simulink model "tqdtqr_rebuild_V3"  (R2021b)
settings: Solver=VariableStepAuto  StartTime=0.0  StopTime=10.0  RelTol=1e-3
undefined symbols (not defined in the file): ATQD_AfterTqMinGain_X_Deg, ATQD_APSCreepBaseTqD_X_kph, ATQD_APSCreepBaseTqD_Y_Deg, ATQD_APSCreepBaseTqR_X_kph, ATQD_APSCreepBaseTqR_Y_Deg, ATQD_APSCreepIterm_X_kph, ATQD_APSCreepIterm_Y_kph, ATQD_APSCreepPterm_X_kph, ATQD_APSCreepPterm_Y_kph, ATQD_APSDecReq_X_kph, ATQD_APSDecReq_Y_mps2, ATQD_APSDecReqCMD_X_kph, ATQD_APSDecReqTs_X_pct, ATQD_APSDecTimeGain_X_Deg, ATQD_APSDecTimeGain_Y_s, ATQD_APSReqLowSpd_X_Deg, ATQD_AutoHoldReleaseBPS_X_Deg, ATQD_AWDLoadTrqnsGain_X_kg, ATQD_AWDLoadTrqnsGain_Y_pct, ATQD_BOSEnBPSPosn_X_kph, ATQD_BOSMap_X_rpm, ATQD_BOSMap_Y_pct, ATQD_CreepBaseTqD_X_kph, ATQD_CreepBaseTqD_Y_Deg, ATQD_CreepBaseTqR_X_kph, ATQD_CreepBaseTqR_Y_Deg, ATQD_CreepBPSDisPosn_X_Deg, ATQD_CreepBPSDisPosnR_X_Deg, ATQD_CreepBPSEnPosn_X_Deg, ATQD_CreepBPSEnPosnR_X_Deg, ATQD_CreepDeltaTq_X_kph, ATQD_CreepIterm_X_kph, ATQD_CreepIterm_Y_kph, ATQD_CreepItermMaxLimit_X_pct, ATQD_CreepPreloadTime_X_kph, ATQD_CreepPreloadTq_X_kph, ATQD_CreepPreloadTq_Y_s, ATQD_CreepProtTq_X_Deg, ATQD_CreepPterm_X_kph, ATQD_CreepPterm_Y_kph, ATQD_CreepRrTqSpRat_X_rpm, ATQD_CreepRrTqSpRat_Y_Nm, ATQD_CreepTargetSpdD_X_pct, ATQD_CreepTargetSpdR_X_pct, ATQD_CreepUpLimitTq_X_rpm, ATQD_DecIneOPDHoldEnDelay_X_Deg, ATQD_DecIneOPDHoldEnDelay_Y_bar, ATQD_ECOTqMapD_X_rpm, ATQD_ECOTqMapD_Y_pct, ATQD_EMTqMapD_X_rpm, ATQD_EMTqMapD_Y_pct, ATQD_EOPDTqMapDCon_X_rpm, ATQD_EOPDTqMapDCon_Y_Deg, ATQD_EstInitVehWeight_X_c, ATQD_FAfterTqCMDGain_X_rpm, ATQD_FAfterTqCMDGain_Y_pct, ATQD_ForceLowSpd_X_Deg, ATQD_ForcePLimitSpd_X_Deg, ATQD_FrLossMAPLowV_X_rpm, ATQD_FrLossMAPLowV_Y_Nm ... (+949)
libraries: simulink x235, hcu_lib x208, tqr x63, tqd x6
(part 34 of 37)

== system tqdtqr_rebuild_V3/Input_Convert/Signal function/combo key/Combo Key Detection/Engineering Mode/Key3/Reset ==
  Action Port : ActionPort  ActionPortLabel=if(u1 ~=0)
  Constant : Constant  Value=ENUM_COMBOKEY_NONE
  ResetToZero : Outport
  wires:
  Constant/1 -> ResetToZero/1

== system tqdtqr_rebuild_V3/Input_Convert/Signal function/combo key/Combo Key Detection/Engineering Mode/Key3/Write ==
  Input : Inport
  Action Port : ActionPort  ActionPortLabel=elseif(u2 ~= 0)
  WriteCMD : Outport
  wires:
  Input/1 -> WriteCMD/1

== system tqdtqr_rebuild_V3/Input_Convert/Signal function/combo key/Combo Key Detection/Engineering Mode/Key4/Maintain ==
  Input : Inport
  Action Port : ActionPort  ActionPortLabel=else
  KeepKey4 : Outport
  wires:
  Input/1 -> KeepKey4/1

== system tqdtqr_rebuild_V3/Input_Convert/Signal function/combo key/Combo Key Detection/Engineering Mode/Key4/Reset ==
  Action Port : ActionPort  ActionPortLabel=if(u1 ~=0)
  Constant : Constant  Value=ENUM_COMBOKEY_NONE
  ResetToZero : Outport
  wires:
  Constant/1 -> ResetToZero/1

== system tqdtqr_rebuild_V3/Input_Convert/Signal function/combo key/Combo Key Detection/Engineering Mode/Key4/Write ==
  Input : Inport
  Action Port : ActionPort  ActionPortLabel=elseif(u2 ~= 0)
  WriteCMD : Outport
  wires:
  Input/1 -> WriteCMD/1

== system tqdtqr_rebuild_V3/Input_Convert/Signal function/combo key/Combo Key Detection/Engineering Mode/Key5/Maintain ==
  Input : Inport
  Action Port : ActionPort  ActionPortLabel=else
  KeepKey5 : Outport
  wires:
  Input/1 -> KeepKey5/1

== system tqdtqr_rebuild_V3/Input_Convert/Signal function/combo key/Combo Key Detection/Engineering Mode/Key5/Reset ==
  Action Port : ActionPort  ActionPortLabel=if(u1 ~=0)
  Constant : Constant  Value=ENUM_COMBOKEY_NONE
  ResetToZero : Outport
  wires:
  Constant/1 -> ResetToZero/1

== system tqdtqr_rebuild_V3/Input_Convert/Signal function/combo key/Combo Key Detection/Engineering Mode/Key5/Write ==
  Input : Inport
  Action Port : ActionPort  ActionPortLabel=elseif(u2 ~= 0)
  WriteCMD : Outport
  wires:
  Input/1 -> WriteCMD/1

== system tqdtqr_rebuild_V3/Input_Convert/Signal function/combo key/Combo Key Detection/Engineering Mode/Key6/Maintain ==
  Input : Inport
  Action Port : ActionPort  ActionPortLabel=else
  KeepKey6 : Outport
  wires:
  Input/1 -> KeepKey6/1

== system tqdtqr_rebuild_V3/Input_Convert/Signal function/combo key/Combo Key Detection/Engineering Mode/Key6/Reset ==
  Action Port : ActionPort  ActionPortLabel=if(u1 ~=0)
  Constant : Constant  Value=ENUM_COMBOKEY_NONE
  ResetToZero : Outport
  wires:
  Constant/1 -> ResetToZero/1

== system tqdtqr_rebuild_V3/Input_Convert/Signal function/combo key/Combo Key Detection/Engineering Mode/Key6/Write ==
  Input : Inport
  Action Port : ActionPort  ActionPortLabel=elseif(u2 ~= 0)
  WriteCMD : Outport
  wires:
  Input/1 -> WriteCMD/1

== system tqdtqr_rebuild_V3/Input_Convert/Signal function/combo key/Combo Key Detection/Engineering Mode/Key7/Maintain ==
  Input : Inport
  Action Port : ActionPort  ActionPortLabel=else
  KeepKey7 : Outport
  wires:
  Input/1 -> KeepKey7/1

== system tqdtqr_rebuild_V3/Input_Convert/Signal function/combo key/Combo Key Detection/Engineering Mode/Key7/Reset ==
  Action Port : ActionPort  ActionPortLabel=if(u1 ~=0)
  Constant : Constant  Value=ENUM_COMBOKEY_NONE
  ResetToZero : Outport
  wires:
  Constant/1 -> ResetToZero/1

== system tqdtqr_rebuild_V3/Input_Convert/Signal function/combo key/Combo Key Detection/Engineering Mode/Key7/Write ==
  Input : Inport
  Action Port : ActionPort  ActionPortLabel=elseif(u2 ~= 0)
  WriteCMD : Outport
  wires:
  Input/1 -> WriteCMD/1

== system tqdtqr_rebuild_V3/Input_Convert/Signal function/combo key/Combo Key Detection/Engineering Mode/Key8/Maintain ==
  Input : Inport
  Action Port : ActionPort  ActionPortLabel=else
  KeepKey8 : Outport
  wires:
  Input/1 -> KeepKey8/1

== system tqdtqr_rebuild_V3/Input_Convert/Signal function/combo key/Combo Key Detection/Engineering Mode/Key8/Reset ==
  Action Port : ActionPort  ActionPortLabel=if(u1 ~=0)
  Constant : Constant  Value=ENUM_COMBOKEY_NONE
  ResetToZero : Outport
  wires:
  Constant/1 -> ResetToZero/1

== system tqdtqr_rebuild_V3/Input_Convert/Signal function/combo key/Combo Key Detection/Engineering Mode/Key8/Write ==
  Input : Inport
  Action Port : ActionPort  ActionPortLabel=elseif(u2 ~= 0)
  WriteCMD : Outport
  wires:
  Input/1 -> WriteCMD/1

== system tqdtqr_rebuild_V3/Input_Convert/Signal function/combo key/Combo Key Detection/Exhibition Mode/Key1/Maintain ==
  Input : Inport
  Action Port : ActionPort  ActionPortLabel=else
  KeepKey1 : Outport
  wires:
  Input/1 -> KeepKey1/1

== system tqdtqr_rebuild_V3/Input_Convert/Signal function/combo key/Combo Key Detection/Exhibition Mode/Key1/Reset ==
  Action Port : ActionPort  ActionPortLabel=if(u1 ~=0)
  Constant : Constant  Value=ENUM_COMBOKEY_NONE
  ResetToZero : Outport
  wires:
  Constant/1 -> ResetToZero/1

== system tqdtqr_rebuild_V3/Input_Convert/Signal function/combo key/Combo Key Detection/Exhibition Mode/Key1/Write ==
  Input : Inport
  Action Port : ActionPort  ActionPortLabel=elseif(u2 ~= 0)
  WriteCMD : Outport
  wires:
  Input/1 -> WriteCMD/1

== system tqdtqr_rebuild_V3/Input_Convert/Signal function/combo key/Combo Key Detection/Exhibition Mode/Key2/Maintain ==
  Input : Inport
  Action Port : ActionPort  ActionPortLabel=else
  KeepKey2 : Outport
  wires:
  Input/1 -> KeepKey2/1

== system tqdtqr_rebuild_V3/Input_Convert/Signal function/combo key/Combo Key Detection/Exhibition Mode/Key2/Reset ==
  Action Port : ActionPort  ActionPortLabel=if(u1 ~=0)
  Constant : Constant  Value=ENUM_COMBOKEY_NONE
  ResetToZero : Outport
  wires:
  Constant/1 -> ResetToZero/1

== system tqdtqr_rebuild_V3/Input_Convert/Signal function/combo key/Combo Key Detection/Exhibition Mode/Key2/Write ==
  Input : Inport
  Action Port : ActionPort  ActionPortLabel=elseif(u2 ~= 0)
  WriteCMD : Outport
  wires:
  Input/1 -> WriteCMD/1

== system tqdtqr_rebuild_V3/Input_Convert/Signal function/combo key/Combo Key Detection/Exhibition Mode/Key3/Maintain ==
  Input : Inport
  Action Port : ActionPort  ActionPortLabel=else
  KeepKey3 : Outport
  wires:
  Input/1 -> KeepKey3/1

== system tqdtqr_rebuild_V3/Input_Convert/Signal function/combo key/Combo Key Detection/Exhibition Mode/Key3/Reset ==
  Action Port : ActionPort  ActionPortLabel=if(u1 ~=0)
  Constant : Constant  Value=ENUM_COMBOKEY_NONE
  ResetToZero : Outport
  wires:
  Constant/1 -> ResetToZero/1

== system tqdtqr_rebuild_V3/Input_Convert/Signal function/combo key/Combo Key Detection/Exhibition Mode/Key3/Write ==
  Input : Inport
  Action Port : ActionPort  ActionPortLabel=elseif(u2 ~= 0)
  WriteCMD : Outport
  wires:
  Input/1 -> WriteCMD/1

== system tqdtqr_rebuild_V3/Input_Convert/Signal function/combo key/Combo Key Detection/Exhibition Mode/Key4/Maintain ==
  Input : Inport
  Action Port : ActionPort  ActionPortLabel=else
  KeepKey4 : Outport
  wires:
  Input/1 -> KeepKey4/1

== system tqdtqr_rebuild_V3/Input_Convert/Signal function/combo key/Combo Key Detection/Exhibition Mode/Key4/Reset ==
  Action Port : ActionPort  ActionPortLabel=if(u1 ~=0)
  Constant : Constant  Value=ENUM_COMBOKEY_NONE
  ResetToZero : Outport
  wires:
  Constant/1 -> ResetToZero/1

== system tqdtqr_rebuild_V3/Input_Convert/Signal function/combo key/Combo Key Detection/Exhibition Mode/Key4/Write ==
  Input : Inport
  Action Port : ActionPort  ActionPortLabel=elseif(u2 ~= 0)
  WriteCMD : Outport
  wires:
  Input/1 -> WriteCMD/1

== system tqdtqr_rebuild_V3/Input_Convert/Signal function/combo key/Combo Key Detection/Exhibition Mode/Key5/Maintain ==
  Input : Inport
  Action Port : ActionPort  ActionPortLabel=else
  KeepKey5 : Outport
  wires:
  Input/1 -> KeepKey5/1

== system tqdtqr_rebuild_V3/Input_Convert/Signal function/combo key/Combo Key Detection/Exhibition Mode/Key5/Reset ==
  Action Port : ActionPort  ActionPortLabel=if(u1 ~=0)
  Constant : Constant  Value=ENUM_COMBOKEY_NONE
  ResetToZero : Outport
  wires:
  Constant/1 -> ResetToZero/1

== system tqdtqr_rebuild_V3/Input_Convert/Signal function/combo key/Combo Key Detection/Exhibition Mode/Key5/Write ==
  Input : Inport
  Action Port : ActionPort  ActionPortLabel=elseif(u2 ~= 0)
  WriteCMD : Outport
  wires:
  Input/1 -> WriteCMD/1

== system tqdtqr_rebuild_V3/Input_Convert/Signal function/combo key/Combo Key Detection/Exhibition Mode/Key6/Maintain ==
  Input : Inport
  Action Port : ActionPort  ActionPortLabel=else
  KeepKey6 : Outport
  wires:
  Input/1 -> KeepKey6/1

== system tqdtqr_rebuild_V3/Input_Convert/Signal function/combo key/Combo Key Detection/Exhibition Mode/Key6/Reset ==
  Action Port : ActionPort  ActionPortLabel=if(u1 ~=0)
  Constant : Constant  Value=ENUM_COMBOKEY_NONE
  ResetToZero : Outport
  wires:
  Constant/1 -> ResetToZero/1

== system tqdtqr_rebuild_V3/Input_Convert/Signal function/combo key/Combo Key Detection/Exhibition Mode/Key6/Write ==
  Input : Inport
  Action Port : ActionPort  ActionPortLabel=elseif(u2 ~= 0)
  WriteCMD : Outport
  wires:
  Input/1 -> WriteCMD/1

== system tqdtqr_rebuild_V3/Input_Convert/Signal function/combo key/Combo Key Detection/Exhibition Mode/Key7/Maintain ==
  Input : Inport
  Action Port : ActionPort  ActionPortLabel=else
  KeepKey7 : Outport
  wires:
  Input/1 -> KeepKey7/1

== system tqdtqr_rebuild_V3/Input_Convert/Signal function/combo key/Combo Key Detection/Exhibition Mode/Key7/Reset ==
  Action Port : ActionPort  ActionPortLabel=if(u1 ~=0)
  Constant : Constant  Value=ENUM_COMBOKEY_NONE
  ResetToZero : Outport
  wires:
  Constant/1 -> ResetToZero/1

== system tqdtqr_rebuild_V3/Input_Convert/Signal function/combo key/Combo Key Detection/Exhibition Mode/Key7/Write ==
  Input : Inport
  Action Port : ActionPort  ActionPortLabel=elseif(u2 ~= 0)
  WriteCMD : Outport
  wires:
  Input/1 -> WriteCMD/1

== system tqdtqr_rebuild_V3/Input_Convert/Signal function/combo key/Combo Key Detection/Exhibition Mode/Key8/Maintain ==
  Input : Inport
  Action Port : ActionPort  ActionPortLabel=else
  KeepKey8 : Outport
  wires:
  Input/1 -> KeepKey8/1

== system tqdtqr_rebuild_V3/Input_Convert/Signal function/combo key/Combo Key Detection/Exhibition Mode/Key8/Reset ==
  Action Port : ActionPort  ActionPortLabel=if(u1 ~=0)
  Constant : Constant  Value=ENUM_COMBOKEY_NONE
  ResetToZero : Outport
  wires:
  Constant/1 -> ResetToZero/1

== system tqdtqr_rebuild_V3/Input_Convert/Signal function/combo key/Combo Key Detection/Exhibition Mode/Key8/Write ==
  Input : Inport
  Action Port : ActionPort  ActionPortLabel=elseif(u2 ~= 0)
  WriteCMD : Outport
  wires:
  Input/1 -> WriteCMD/1

== system tqdtqr_rebuild_V3/Input_Convert/Signal function/combo key/Combo Key Detection/Manufacture Mode/Key1/Maintain ==
  Input : Inport
  Action Port : ActionPort  ActionPortLabel=else
  KeepKey1 : Outport
  wires:
  Input/1 -> KeepKey1/1

== system tqdtqr_rebuild_V3/Input_Convert/Signal function/combo key/Combo Key Detection/Manufacture Mode/Key1/Reset ==
  Action Port : ActionPort  ActionPortLabel=if(u1 ~=0)
  Constant : Constant  Value=ENUM_COMBOKEY_NONE
  ResetToZero : Outport
  wires:
  Constant/1 -> ResetToZero/1

== system tqdtqr_rebuild_V3/Input_Convert/Signal function/combo key/Combo Key Detection/Manufacture Mode/Key1/Write ==
  Input : Inport
  Action Port : ActionPort  ActionPortLabel=elseif(u2 ~= 0)
  WriteCMD : Outport
  wires:
  Input/1 -> WriteCMD/1

== system tqdtqr_rebuild_V3/Input_Convert/Signal function/combo key/Combo Key Detection/Manufacture Mode/Key2/Maintain ==
  Input : Inport
  Action Port : ActionPort  ActionPortLabel=else
  KeepKey2 : Outport
  wires:
  Input/1 -> KeepKey2/1

== system tqdtqr_rebuild_V3/Input_Convert/Signal function/combo key/Combo Key Detection/Manufacture Mode/Key2/Reset ==
  Action Port : ActionPort  ActionPortLabel=if(u1 ~=0)
  Constant : Constant  Value=ENUM_COMBOKEY_NONE
  ResetToZero : Outport
  wires:
  Constant/1 -> ResetToZero/1

== system tqdtqr_rebuild_V3/Input_Convert/Signal function/combo key/Combo Key Detection/Manufacture Mode/Key2/Write ==
  Input : Inport
  Action Port : ActionPort  ActionPortLabel=elseif(u2 ~= 0)
  WriteCMD : Outport
  wires:
  Input/1 -> WriteCMD/1

== system tqdtqr_rebuild_V3/Input_Convert/Signal function/combo key/Combo Key Detection/Manufacture Mode/Key3/Maintain ==
  Input : Inport
  Action Port : ActionPort  ActionPortLabel=else
  KeepKey3 : Outport
  wires:
  Input/1 -> KeepKey3/1

== system tqdtqr_rebuild_V3/Input_Convert/Signal function/combo key/Combo Key Detection/Manufacture Mode/Key3/Reset ==
  Action Port : ActionPort  ActionPortLabel=if(u1 ~=0)
  Constant : Constant  Value=ENUM_COMBOKEY_NONE
  ResetToZero : Outport
  wires:
  Constant/1 -> ResetToZero/1

== system tqdtqr_rebuild_V3/Input_Convert/Signal function/combo key/Combo Key Detection/Manufacture Mode/Key3/Write ==
  Input : Inport
  Action Port : ActionPort  ActionPortLabel=elseif(u2 ~= 0)
  WriteCMD : Outport
  wires:
  Input/1 -> WriteCMD/1

== system tqdtqr_rebuild_V3/Input_Convert/Signal function/combo key/Combo Key Detection/Manufacture Mode/Key4/Maintain ==
  Input : Inport
  Action Port : ActionPort  ActionPortLabel=else
  KeepKey4 : Outport
  wires:
  Input/1 -> KeepKey4/1

== system tqdtqr_rebuild_V3/Input_Convert/Signal function/combo key/Combo Key Detection/Manufacture Mode/Key4/Reset ==
  Action Port : ActionPort  ActionPortLabel=if(u1 ~=0)
  Constant : Constant  Value=ENUM_COMBOKEY_NONE
  ResetToZero : Outport
  wires:
  Constant/1 -> ResetToZero/1

== system tqdtqr_rebuild_V3/Input_Convert/Signal function/combo key/Combo Key Detection/Manufacture Mode/Key4/Write ==
  Input : Inport
  Action Port : ActionPort  ActionPortLabel=elseif(u2 ~= 0)
  WriteCMD : Outport
  wires:
  Input/1 -> WriteCMD/1

== system tqdtqr_rebuild_V3/Input_Convert/Signal function/combo key/Combo Key Detection/Manufacture Mode/Key5/Maintain ==
  Input : Inport
  Action Port : ActionPort  ActionPortLabel=else
  KeepKey5 : Outport
  wires:
  Input/1 -> KeepKey5/1

== system tqdtqr_rebuild_V3/Input_Convert/Signal function/combo key/Combo Key Detection/Manufacture Mode/Key5/Reset ==
  Action Port : ActionPort  ActionPortLabel=if(u1 ~=0)
  Constant : Constant  Value=ENUM_COMBOKEY_NONE
  ResetToZero : Outport
  wires:
  Constant/1 -> ResetToZero/1

== system tqdtqr_rebuild_V3/Input_Convert/Signal function/combo key/Combo Key Detection/Manufacture Mode/Key5/Write ==
  Input : Inport
  Action Port : ActionPort  ActionPortLabel=elseif(u2 ~= 0)
  WriteCMD : Outport
  wires:
  Input/1 -> WriteCMD/1

== system tqdtqr_rebuild_V3/Input_Convert/Signal function/combo key/Combo Key Detection/Manufacture Mode/Key6/Maintain ==
  Input : Inport
  Action Port : ActionPort  ActionPortLabel=else
  KeepKey6 : Outport
  wires:
  Input/1 -> KeepKey6/1

== system tqdtqr_rebuild_V3/Input_Convert/Signal function/combo key/Combo Key Detection/Manufacture Mode/Key6/Reset ==
  Action Port : ActionPort  ActionPortLabel=if(u1 ~=0)
  Constant : Constant  Value=ENUM_COMBOKEY_NONE
  ResetToZero : Outport
  wires:
  Constant/1 -> ResetToZero/1

== system tqdtqr_rebuild_V3/Input_Convert/Signal function/combo key/Combo Key Detection/Manufacture Mode/Key6/Write ==
  Input : Inport
  Action Port : ActionPort  ActionPortLabel=elseif(u2 ~= 0)
  WriteCMD : Outport
  wires:
  Input/1 -> WriteCMD/1

== system tqdtqr_rebuild_V3/Input_Convert/Signal function/combo key/Combo Key Detection/Manufacture Mode/Key7/Maintain ==
  Input : Inport
  Action Port : ActionPort  ActionPortLabel=else
  KeepKey7 : Outport
  wires:
  Input/1 -> KeepKey7/1

== system tqdtqr_rebuild_V3/Input_Convert/Signal function/combo key/Combo Key Detection/Manufacture Mode/Key7/Reset ==
  Action Port : ActionPort  ActionPortLabel=if(u1 ~=0)
  Constant : Constant  Value=ENUM_COMBOKEY_NONE
  ResetToZero : Outport
  wires:
  Constant/1 -> ResetToZero/1

== system tqdtqr_rebuild_V3/Input_Convert/Signal function/combo key/Combo Key Detection/Manufacture Mode/Key7/Write ==
  Input : Inport
  Action Port : ActionPort  ActionPortLabel=elseif(u2 ~= 0)
  WriteCMD : Outport
  wires:
  Input/1 -> WriteCMD/1

== system tqdtqr_rebuild_V3/Input_Convert/Signal function/combo key/Combo Key Detection/Manufacture Mode/Key8/Maintain ==
  Input : Inport
  Action Port : ActionPort  ActionPortLabel=else
  KeepKey8 : Outport
  wires:
  Input/1 -> KeepKey8/1

== system tqdtqr_rebuild_V3/Input_Convert/Signal function/combo key/Combo Key Detection/Manufacture Mode/Key8/Reset ==
  Action Port : ActionPort  ActionPortLabel=if(u1 ~=0)
  Constant : Constant  Value=ENUM_COMBOKEY_NONE
  ResetToZero : Outport
  wires:
  Constant/1 -> ResetToZero/1

== system tqdtqr_rebuild_V3/Input_Convert/Signal function/combo key/Combo Key Detection/Manufacture Mode/Key8/Write ==
  Input : Inport
  Action Port : ActionPort  ActionPortLabel=elseif(u2 ~= 0)
  WriteCMD : Outport
  wires:
  Input/1 -> WriteCMD/1

== system tqdtqr_rebuild_V3/Input_Convert/Signal function/combo key/Combo Key Detection/Street Fight Mode/Key1/Maintain ==
  Input : Inport
  Action Port : ActionPort  ActionPortLabel=else
  KeepKey1 : Outport
  wires:
  Input/1 -> KeepKey1/1

== system tqdtqr_rebuild_V3/Input_Convert/Signal function/combo key/Combo Key Detection/Street Fight Mode/Key1/Reset ==
  Action Port : ActionPort  ActionPortLabel=if(u1 ~=0)
  Constant : Constant  Value=ENUM_COMBOKEY_NONE
  ResetToZero : Outport
  wires:
  Constant/1 -> ResetToZero/1

== system tqdtqr_rebuild_V3/Input_Convert/Signal function/combo key/Combo Key Detection/Street Fight Mode/Key1/Write ==
  Input : Inport
  Action Port : ActionPort  ActionPortLabel=elseif(u2 ~= 0)
  WriteCMD : Outport
  wires:
  Input/1 -> WriteCMD/1

== system tqdtqr_rebuild_V3/Input_Convert/Signal function/combo key/Combo Key Detection/Street Fight Mode/Key2/Maintain ==
  Input : Inport
  Action Port : ActionPort  ActionPortLabel=else
  KeepKey2 : Outport
  wires:
  Input/1 -> KeepKey2/1

== system tqdtqr_rebuild_V3/Input_Convert/Signal function/combo key/Combo Key Detection/Street Fight Mode/Key2/Reset ==
  Action Port : ActionPort  ActionPortLabel=if(u1 ~=0)
  Constant : Constant  Value=ENUM_COMBOKEY_NONE
  ResetToZero : Outport
  wires:
  Constant/1 -> ResetToZero/1

== system tqdtqr_rebuild_V3/Input_Convert/Signal function/combo key/Combo Key Detection/Street Fight Mode/Key2/Write ==
  Input : Inport
  Action Port : ActionPort  ActionPortLabel=elseif(u2 ~= 0)
  WriteCMD : Outport
  wires:
  Input/1 -> WriteCMD/1

== system tqdtqr_rebuild_V3/Input_Convert/Signal function/combo key/Combo Key Detection/Street Fight Mode/Key3/Maintain ==
  Input : Inport
  Action Port : ActionPort  ActionPortLabel=else
  KeepKey3 : Outport
  wires:
  Input/1 -> KeepKey3/1

== system tqdtqr_rebuild_V3/Input_Convert/Signal function/combo key/Combo Key Detection/Street Fight Mode/Key3/Reset ==
  Action Port : ActionPort  ActionPortLabel=if(u1 ~=0)
  Constant : Constant  Value=ENUM_COMBOKEY_NONE
  ResetToZero : Outport
  wires:
  Constant/1 -> ResetToZero/1

== system tqdtqr_rebuild_V3/Input_Convert/Signal function/combo key/Combo Key Detection/Street Fight Mode/Key3/Write ==
  Input : Inport
  Action Port : ActionPort  ActionPortLabel=elseif(u2 ~= 0)
  WriteCMD : Outport
  wires:
  Input/1 -> WriteCMD/1

== system tqdtqr_rebuild_V3/Input_Convert/Signal function/combo key/Combo Key Detection/Street Fight Mode/Key4/Maintain ==
  Input : Inport
  Action Port : ActionPort  ActionPortLabel=else
  KeepKey4 : Outport
  wires:
  Input/1 -> KeepKey4/1

== system tqdtqr_rebuild_V3/Input_Convert/Signal function/combo key/Combo Key Detection/Street Fight Mode/Key4/Reset ==
  Action Port : ActionPort  ActionPortLabel=if(u1 ~=0)
  Constant : Constant  Value=ENUM_COMBOKEY_NONE
  ResetToZero : Outport
  wires:
  Constant/1 -> ResetToZero/1

== system tqdtqr_rebuild_V3/Input_Convert/Signal function/combo key/Combo Key Detection/Street Fight Mode/Key4/Write ==
  Input : Inport
  Action Port : ActionPort  ActionPortLabel=elseif(u2 ~= 0)
  WriteCMD : Outport
  wires:
  Input/1 -> WriteCMD/1

== system tqdtqr_rebuild_V3/Input_Convert/Signal function/combo key/Combo Key Detection/Street Fight Mode/Key5/Maintain ==
  Input : Inport
  Action Port : ActionPort  ActionPortLabel=else
  KeepKey5 : Outport
  wires:
  Input/1 -> KeepKey5/1

== system tqdtqr_rebuild_V3/Input_Convert/Signal function/combo key/Combo Key Detection/Street Fight Mode/Key5/Reset ==
  Action Port : ActionPort  ActionPortLabel=if(u1 ~=0)
  Constant : Constant  Value=ENUM_COMBOKEY_NONE
  ResetToZero : Outport
  wires:
  Constant/1 -> ResetToZero/1

== system tqdtqr_rebuild_V3/Input_Convert/Signal function/combo key/Combo Key Detection/Street Fight Mode/Key5/Write ==
  Input : Inport
  Action Port : ActionPort  ActionPortLabel=elseif(u2 ~= 0)
  WriteCMD : Outport
  wires:
  Input/1 -> WriteCMD/1

== system tqdtqr_rebuild_V3/Input_Convert/Signal function/combo key/Combo Key Detection/Street Fight Mode/Key6/Maintain ==
  Input : Inport
  Action Port : ActionPort  ActionPortLabel=else
  KeepKey6 : Outport
  wires:
  Input/1 -> KeepKey6/1

== system tqdtqr_rebuild_V3/Input_Convert/Signal function/combo key/Combo Key Detection/Street Fight Mode/Key6/Reset ==
  Action Port : ActionPort  ActionPortLabel=if(u1 ~=0)
  Constant : Constant  Value=ENUM_COMBOKEY_NONE
  ResetToZero : Outport
  wires:
  Constant/1 -> ResetToZero/1

== system tqdtqr_rebuild_V3/Input_Convert/Signal function/combo key/Combo Key Detection/Street Fight Mode/Key6/Write ==
  Input : Inport
  Action Port : ActionPort  ActionPortLabel=elseif(u2 ~= 0)
  WriteCMD : Outport
  wires:
  Input/1 -> WriteCMD/1

== system tqdtqr_rebuild_V3/Input_Convert/Signal function/combo key/Combo Key Detection/Street Fight Mode/Key7/Maintain ==
  Input : Inport
  Action Port : ActionPort  ActionPortLabel=else
  KeepKey7 : Outport
  wires:
  Input/1 -> KeepKey7/1

== system tqdtqr_rebuild_V3/Input_Convert/Signal function/combo key/Combo Key Detection/Street Fight Mode/Key7/Reset ==
  Action Port : ActionPort  ActionPortLabel=if(u1 ~=0)
  Constant : Constant  Value=ENUM_COMBOKEY_NONE
  ResetToZero : Outport
  wires:
  Constant/1 -> ResetToZero/1

== system tqdtqr_rebuild_V3/Input_Convert/Signal function/combo key/Combo Key Detection/Street Fight Mode/Key7/Write ==
  Input : Inport
  Action Port : ActionPort  ActionPortLabel=elseif(u2 ~= 0)
  WriteCMD : Outport
  wires:
  Input/1 -> WriteCMD/1

== system tqdtqr_rebuild_V3/Input_Convert/Signal function/combo key/Combo Key Detection/Street Fight Mode/Key8/Maintain ==
  Input : Inport
  Action Port : ActionPort  ActionPortLabel=else
  KeepKey8 : Outport
  wires:
  Input/1 -> KeepKey8/1

== system tqdtqr_rebuild_V3/Input_Convert/Signal function/combo key/Combo Key Detection/Street Fight Mode/Key8/Reset ==
  Action Port : ActionPort  ActionPortLabel=if(u1 ~=0)
  Constant : Constant  Value=ENUM_COMBOKEY_NONE
  ResetToZero : Outport
  wires:
  Constant/1 -> ResetToZero/1

== system tqdtqr_rebuild_V3/Input_Convert/Signal function/combo key/Combo Key Detection/Street Fight Mode/Key8/Write ==
  Input : Inport
  Action Port : ActionPort  ActionPortLabel=elseif(u2 ~= 0)
  WriteCMD : Outport
  wires:
  Input/1 -> WriteCMD/1

== stateflow chart tqdtqr_rebuild_V3/Input_Convert/Main function/DriverWhlTqDem function/Driver mode determination/Pedal map conditions decide ==
  (default) -> (junction 3)
  (junction 3) -> (junction 5) [order 1] : [(VTQD_LimpHomeAct_flg && KTQD_FailsafeActiveSW_flg) || ~VTQD_EVDriveModeValid_flg]
  (junction 3) -> (junction 9) [order 2]
  (junction 5) -> (junction 7) : {VTQD_PedalMapAction_enum = ENUM_PEDALMAPACTION_LHM;}
  (junction 9) -> (junction 11) [order 1] : [VTQD_GearActualPosn_enum==ENUM_GEARACTUALPOSN_R]
  (junction 9) -> (junction 16) [order 2]
  (junction 11) -> (junction 34) : {VTQD_PedalMapAction_enum = ENUM_PEDALMAPACTION_NOLHMR;}
  (junction 16) -> (junction 19) [order 1] : [VTQD_GearActualPosn_enum==ENUM_GEARACTUALPOSN_D]
  (junction 19) -> (junction 26) [order 1] : [VTQD_IVIRockModeEn_flg]
  (junction 16) -> (junction 24) [order 2] : {VTQD_PedalMapAction_enum = ENUM_PEDALMAPACTION_NOLHMN;}
  (junction 19) -> (junction 65) [order 2]
  (junction 26) -> (junction 63) : {VTQD_PedalMapAction_enum =ENUM_PEDALMAPACTION_NOLHMDROCK;}
  (junction 65) -> (junction 67) [order 1] : [VINP_IVISnowModeCmd_flg]
  (junction 65) -> (junction 71) [order 2]
  (junction 67) -> (junction 69) : {VTQD_PedalMapAction_enum = ENUM_PEDALMAPACTION_NOLHMDSNOW;}
  (junction 71) -> (junction 73) [order 1] : [VTQD_EVDriveMode_enum==ENUM_DRIVEMODE_NRM]
  (junction 73) -> (junction 93) [order 1] : [VTQD_RegenMode_enum==ENUM_REGENLEVEL_LV1]
  (junction 71) -> (junction 77) [order 2]
  (junction 73) -> (junction 95) [order 2]
  (junction 93) -> (junction 75) : {VTQD_PedalMapAction_enum = ENUM_PEDALMAPACTION_NOLHMDNRMLV1;}
  (junction 95) -> (junction 97) [order 1] : [VTQD_RegenMode_enum==ENUM_REGENLEVEL_LV2]
  (junction 95) -> (junction 101) [order 2]
  (junction 97) -> (junction 99) : {VTQD_PedalMapAction_enum = ENUM_PEDALMAPACTION_NOLHMDNRMLV2;}
  (junction 101) -> (junction 103) [order 1] : [VTQD_RegenMode_enum==ENUM_REGENLEVEL_LV3]
  (junction 101) -> (junction 106) [order 2]
  (junction 103) -> (junction 113) : {VTQD_PedalMapAction_enum = ENUM_PEDALMAPACTION_NOLHMDNRMLV3;}
  (junction 106) -> (junction 107) [order 1] : [VTQD_RegenMode_enum==ENUM_REGENLEVEL_LV4]
  (junction 106) -> (junction 110) [order 2]
  (junction 107) -> (junction 115) : {VTQD_PedalMapAction_enum = ENUM_PEDALMAPACTION_NOLHMDNRMLV4;}
  (junction 110) -> (junction 111) [order 1] : [VTQD_RegenMode_enum==ENUM_REGENLEVEL_LV5]
  (junction 110) -> (junction 159) [order 2]
  (junction 111) -> (junction 117) : {VTQD_PedalMapAction_enum = ENUM_PEDALMAPACTION_NOLHMDNRMLV5;}
  (junction 159) -> (junction 157) [order 1] : [VTQD_RegenMode_enum==ENUM_REGENLEVEL_OPD]
  (junction 159) -> (junction 199) [order 2] : {VTQD_PedalMapAction_enum = ENUM_PEDALMAPACTION_NOLHMDNRMINV;}
  (junction 157) -> (junction 158) : {VTQD_PedalMapAction_enum = ENUM_PEDALMAPACTION_NOLHMDNRMOPD;}
  (junction 77) -> (junction 79) [order 1] : [VTQD_EVDriveMode_enum==ENUM_DRIVEMODE_ECO]
  (junction 79) -> (junction 119) [order 1] : [VTQD_RegenMode_enum==ENUM_REGENLEVEL_LV1]
  (junction 77) -> (junction 83) [order 2]
  (junction 79) -> (junction 126) [order 2]
  (junction 119) -> (junction 81) : {VTQD_PedalMapAction_enum = ENUM_PEDALMAPACTION_NOLHMDECOLV1;}
  (junction 126) -> (junction 128) [order 1] : [VTQD_RegenMode_enum==ENUM_REGENLEVEL_LV2]
  (junction 126) -> (junction 136) [order 2]
  (junction 128) -> (junction 130) : {VTQD_PedalMapAction_enum = ENUM_PEDALMAPACTION_NOLHMDECOLV2;}
  (junction 136) -> (junction 135) [order 1] : [VTQD_RegenMode_enum==ENUM_REGENLEVEL_LV3]
  (junction 136) -> (junction 141) [order 2]
  (junction 135) -> (junction 132) : {VTQD_PedalMapAction_enum = ENUM_PEDALMAPACTION_NOLHMDECOLV3;}
  (junction 141) -> (junction 140) [order 1] : [VTQD_RegenMode_enum==ENUM_REGENLEVEL_LV4]
  (junction 141) -> (junction 147) [order 2]
  (junction 140) -> (junction 138) : {VTQD_PedalMapAction_enum = ENUM_PEDALMAPACTION_NOLHMDECOLV4;}
  (junction 147) -> (junction 146) [order 1] : [VTQD_RegenMode_enum==ENUM_REGENLEVEL_LV5]
  (junction 147) -> (junction 153) [order 2]
  (junction 146) -> (junction 144) : {VTQD_PedalMapAction_enum = ENUM_PEDALMAPACTION_NOLHMDECOLV5;}
  (junction 153) -> (junction 152) [order 1] : [VTQD_RegenMode_enum==ENUM_REGENLEVEL_OPD]
  (junction 153) -> (junction 197) [order 2] : {VTQD_PedalMapAction_enum = ENUM_PEDALMAPACTION_NOLHMDECOINV;}
  (junction 152) -> (junction 150) : {VTQD_PedalMapAction_enum = ENUM_PEDALMAPACTION_NOLHMDECOOPD;}
  (junction 85) -> (junction 163) [order 1] : [VTQD_RegenMode_enum==ENUM_REGENLEVEL_LV1]
  (junction 83) -> (junction 85) : [VTQD_EVDriveMode_enum==ENUM_DRIVEMODE_SPORT]
  (junction 163) -> (junction 87) : {VTQD_PedalMapAction_enum = ENUM_PEDALMAPACTION_NOLHMDSPORTLV1;}
  (junction 85) -> (junction 165) [order 2]
  (junction 165) -> (junction 167) [order 1] : [VTQD_RegenMode_enum==ENUM_REGENLEVEL_LV2]
  (junction 165) -> (junction 176) [order 2]
  (junction 167) -> (junction 169) : {VTQD_PedalMapAction_enum = ENUM_PEDALMAPACTION_NOLHMDSPORTLV2;}
  (junction 176) -> (junction 172) [order 1] : [VTQD_RegenMode_enum==ENUM_REGENLEVEL_LV3]
  (junction 176) -> (junction 177) [order 2]
  (junction 172) -> (junction 175) : {VTQD_PedalMapAction_enum = ENUM_PEDALMAPACTION_NOLHMDSPORTLV3;}
  (junction 177) -> (junction 179) [order 1] : [VTQD_RegenMode_enum==ENUM_REGENLEVEL_LV4]
  (junction 177) -> (junction 183) [order 2]
  (junction 179) -> (junction 182) : {VTQD_PedalMapAction_enum = ENUM_PEDALMAPACTION_NOLHMDSPORTLV4;}
  (junction 183) -> (junction 185) [order 1] : [VTQD_RegenMode_enum==ENUM_REGENLEVEL_LV5]
  (junction 183) -> (junction 189) [order 2]
  (junction 185) -> (junction 188) : {VTQD_PedalMapAction_enum = ENUM_PEDALMAPACTION_NOLHMDSPORTLV5;}
  (junction 189) -> (junction 191) [order 1] : [VTQD_RegenMode_enum==ENUM_REGENLEVEL_OPD]
  (junction 189) -> (junction 195) [order 2] : {VTQD_PedalMapAction_enum = ENUM_PEDALMAPACTION_NOLHMDSPORTINV;}
  (junction 191) -> (junction 194) : {VTQD_PedalMapAction_enum = ENUM_PEDALMAPACTION_NOLHMDSPORTOPD;}
  data: VTQD_LimpHomeAct_flg input; VTQD_EVDriveModeValid_flg input; KTQD_FailsafeActiveSW_flg parameter; VTQD_PedalMapAction_enum output uint8; VTQD_GearActualPosn_enum input; ENUM_GEARACTUALPOSN_D parameter; ENUM_GEARACTUALPOSN_R parameter; VTQD_IVIRockModeEn_flg input; VINP_IVISnowModeCmd_flg input; VTQD_EVDriveMode_enum input; ENUM_DRIVEMODE_NRM parameter; ENUM_DRIVEMODE_ECO parameter; ENUM_DRIVEMODE_SPORT parameter; VTQD_RegenMode_enum input; ENUM_REGENLEVEL_LV1 parameter; ENUM_REGENLEVEL_LV2 parameter; ENUM_REGENLEVEL_LV3 parameter; ENUM_REGENLEVEL_LV4 parameter; ENUM_REGENLEVEL_LV5 parameter; ENUM_REGENLEVEL_OPD parameter; ENUM_PEDALMAPACTION_LHM parameter; ENUM_PEDALMAPACTION_NOLHMDROCK parameter; ENUM_PEDALMAPACTION_NOLHMR parameter; ENUM_PEDALMAPACTION_NOLHMN parameter; ENUM_PEDALMAPACTION_NOLHMDNRMLV5 parameter; ENUM_PEDALMAPACTION_NOLHMDNRMLV3 parameter; ENUM_PEDALMAPACTION_NOLHMDNRMLV4 parameter; ENUM_PEDALMAPACTION_NOLHMDNRMOPD parameter; ENUM_PEDALMAPACTION_NOLHMDSNOW parameter; ENUM_PEDALMAPACTION_NOLHMDNRMLV1 parameter; ENUM_PEDALMAPACTION_NOLHMDNRMLV2 parameter; ENUM_PEDALMAPACTION_NOLHMDSPORTLV1 parameter; ENUM_PEDALMAPACTION_NOLHMDECOLV1 parameter; ENUM_PEDALMAPACTION_NOLHMDECOLV3 parameter; ENUM_PEDALMAPACTION_NOLHMDECOLV5 parameter; ENUM_PEDALMAPACTION_NOLHMDECOLV2 parameter; ENUM_PEDALMAPACTION_NOLHMDECOLV4 parameter; ENUM_PEDALMAPACTION_NOLHMDECOOPD parameter; ENUM_PEDALMAPACTION_NOLHMDSPORTLV2 parameter; ENUM_PEDALMAPACTION_NOLHMDSPORTOPD parameter; ENUM_PEDALMAPACTION_NOLHMDSPORTLV4 parameter; ENUM_PEDALMAPACTION_NOLHMDECOINV parameter; ENUM_PEDALMAPACTION_NOLHMDSPORTLV3 parameter; ENUM_PEDALMAPACTION_NOLHMDSPORTLV5 parameter; ENUM_PEDALMAPACTION_NOLHMDNRMINV parameter; ENUM_PEDALMAPACTION_NOLHMDSPORTINV parameter

== stateflow chart tqdtqr_rebuild_V3/Input_Convert/Signal function/ShiftModule/Determine_Actual_Gear_Position ==
  state P
    en:
    VTQD_GearActualPosn_enum = ENUM_GEARACTUALPOSN_P;
    VTQD_ParkRequest_flg = TRUE;
    VTQD_ExitP_flg = FALSE;
    (default) -> (junction 636) : {
        | VTQD_ReunlockWaitTime_s = 0;
        | }
    P -> (junction 636) [order 1]
    (junction 636) -> (junction 641) [order 1] : %[!VTQD_PBWUnlockTO_flg]
    (junction 636) -> (junction 645) [order 2] : {
        | VTQD_ReunlockWaitTime_s += task_time_s;
        | }
    (junction 641) -> (junction 637) : {
        | VTQD_ExitP_flg = TRUE;
        | }
    (junction 645) -> (junction 632) [order 1] : [VTQD_ReunlockWaitTime_s >= KTQD_ReunlockWaitTime_s]
    (junction 645) -> (junction 647) [order 2]
    (junction 632) -> (junction 643) : {
        | VTQD_ExitP_flg = TRUE;
        | }
    (junction 643) -> (junction 647)
    (junction 637) -> (junction 643)
  state N
    en:
    VTQD_GearActualPosn_enum = ENUM_GEARACTUALPOSN_N;
    VTQD_ParkRequest_flg = FALSE;
    VTQD_EnterP_flg = FALSE;
    (default) -> (junction 753) : {
        | VTQD_RelockWaitTime_s = 0;
        | }
    (junction 753) -> (junction 754) [order 1] : %[!VTQD_PBWLockTO_flg]
    N -> (junction 753) [order 1]
    (junction 753) -> (junction 755) [order 2] : {
        | VTQD_RelockWaitTime_s += task_time_s;
        | }
    (junction 754) -> (junction 757) : {
        | VTQD_EnterP_flg = TRUE;
        | }
    (junction 755) -> (junction 756) [order 1] : [VTQD_RelockWaitTime_s >= KTQD_RelockWaitTime_s]
    (junction 755) -> (junction 760) [order 2]
    (junction 756) -> (junction 758) : {
        | VTQD_EnterP_flg = TRUE;
        | }
    (junction 758) -> (junction 760)
    (junction 757) -> (junction 758)
  state D
    en:
    VTQD_GearActualPosn_enum = ENUM_GEARACTUALPOSN_D;
    VTQD_ParkRequest_flg = FALSE;
  state R
    en:
    VTQD_GearActualPosn_enum = ENUM_GEARACTUALPOSN_R;
    VTQD_ParkRequest_flg = FALSE;
  (default) -> P : {
      |  VTQD_PBWLockTO_flg = FALSE;
      |  VTQD_PBWUnlockTO_flg = FALSE;
      | }
  P -> N [order 1] : [VTQD_GearP2N_flg]
  N -> (junction 731) [order 2] : [VTQD_GearN2R_flg]
  (junction 731) -> (junction 733)
  N -> P [order 3] : [VTQD_GearN2P_flg]
  (junction 749) -> N
  (junction 747) -> (junction 749)
  D -> N [order 1] : [VTQD_GearD2N_flg]
  N -> D [order 1] : [VTQD_GearN2D_flg]
  P -> D [order 2] : [VTQD_GearP2D_flg]
  D -> P [order 2] : [VTQD_GearD2P_flg]
  R -> D [order 3] : [VTQD_GearR2D_flg]
  D -> R [order 3] : [VTQD_GearD2R_flg]
  P -> R [order 3] : [VTQD_GearP2R_flg]
  R -> (junction 747) [order 1] : [VTQD_GearR2N_flg]
  (junction 733) -> R
  R -> P [order 2] : [VTQD_GearR2P_flg]
  data: task_time_s input; VTQD_GearActualPosn_enum output uint8; ENUM_GEARACTUALPOSN_N parameter; ENUM_GEARACTUALPOSN_D parameter; ENUM_GEARACTUALPOSN_R parameter; ENUM_GEARACTUALPOSN_P parameter; FALSE parameter; TRUE parameter; VTQD_PBWLockTO_flg output boolean; VTQD_PBWUnlockTO_flg output boolean; VTQD_ParkRequest_flg output boolean; VTQD_RelockWaitTime_s local single; VTQD_ReunlockWaitTime_s local single; VTQD_GearP2N_flg input; VTQD_GearN2P_flg input; VTQD_GearP2D_flg input; VTQD_GearD2P_flg input; VTQD_GearP2R_flg input; VTQD_GearR2P_flg input; VTQD_GearN2D_flg input; VTQD_GearD2N_flg input; VTQD_GearD2R_flg input; VTQD_GearR2D_flg input; VTQD_GearN2R_flg input; VTQD_GearR2N_flg input; VTQD_ExitP_flg output boolean; VTQD_EnterP_flg output boolean; KTQD_RelockWaitTime_s parameter; KTQD_ReunlockWaitTime_s parameter

== stateflow chart tqdtqr_rebuild_V3/Input_Convert/Signal function/SWC1 SWC2 status/SWC2_Subsystem/Speed Control Mode ==
  state OFF
    en:
    VTQD_SpdCtrlMode_enum = ENUM_SPDCTRLMODE_OFF;
    VTQD_SpdCtrlSta_flg = FALSE;
  state ACC
    en:
    VTQD_SpdCtrlMode_enum = ENUM_SPDCTRLMODE_ACC;
    VTQD_SpdCtrlSta_flg = TRUE;
  state MSA
    en:
    VTQD_SpdCtrlMode_enum = ENUM_SPDCTRLMODE_MSA;
    VTQD_SpdCtrlSta_flg = TRUE;
  (default) -> OFF
  (junction 117) -> OFF
  (junction 26) -> (junction 117) [order 1] : [
      |  VPMM_PowerSta_enum != ENUM_POWERSTA_READY || ...
      |  VTQD_ShiftGearPosn_enum == ENUM_GEARPOSNTOCAN_P
      | ]
  ACC -> OFF [order 1] : [
      | VPMM_PowerSta_enum != ENUM_POWERSTA_READY || ...
      | VTQD_ShiftGearPosn_enum != ENUM_GEARPOSNTOCAN_D
      | ]
  OFF -> ACC : [
      | VPMM_PowerSta_enum == ENUM_POWERSTA_READY && ...
      | VTQD_ShiftGearPosn_enum == ENUM_GEARPOSNTOCAN_D
      | ]
  (junction 26) -> ACC [order 2]
  (junction 19) -> (junction 26)
  ACC -> MSA [order 2] : [VTQD_LScrollPressLong_flg && ...
      | VVMC_MSACtrlSta_enum != ENUM_ADASMSASTA_ACTIVE]
      | %add20241210
  MSA -> (junction 19) : [
      |  VPMM_PowerSta_enum != ENUM_POWERSTA_READY || ...
      |  VTQD_ShiftGearPosn_enum == ENUM_GEARPOSNTOCAN_P ||...
      |  VTQD_SWC2LADASSta_flg
      |  ]
      | %add20241210
  data: VPMM_PowerSta_enum input; VTQD_LScrollPressLong_flg input; ENUM_SPDCTRLMODE_OFF parameter; ENUM_SPDCTRLMODE_ACC parameter; ENUM_SPDCTRLMODE_MSA parameter; FALSE parameter; ENUM_POWERSTA_READY parameter; VTQD_SpdCtrlMode_enum output uint8; VTQD_SpdCtrlSta_flg output boolean; TRUE parameter; VTQD_ShiftGearPosn_enum input; ENUM_GEARPOSNTOCAN_D parameter; ENUM_GEARPOSNTOCAN_P parameter; VTQD_SWC2LADASSta_flg input; VVMC_MSACtrlSta_enum input; ENUM_ADASMSASTA_ACTIVE parameter

== stateflow chart tqdtqr_rebuild_V3/Input_Convert/Signal function/Regen level define/Regen Level Switch ==
  state OFF
    en:
    VTQD_RegenMode_enum = ENUM_REGENLEVEL_OFF;
  state UserSetting
  state Lv1
    en:
    VTQD_RegenMode_enum = ENUM_REGENLEVEL_LV1;
    VTQD_SaveRegenMode_enum = ENUM_REGENLEVEL_LV1;
  state Lv2
    en:
    VTQD_RegenMode_enum = ENUM_REGENLEVEL_LV2;
    VTQD_SaveRegenMode_enum = ENUM_REGENLEVEL_LV2;
  state Lv3
    en:
    VTQD_RegenMode_enum = ENUM_REGENLEVEL_LV3;
    VTQD_SaveRegenMode_enum = ENUM_REGENLEVEL_LV3;
  state Lv4
    en:
    VTQD_RegenMode_enum = ENUM_REGENLEVEL_LV4;
    VTQD_SaveRegenMode_enum = ENUM_REGENLEVEL_LV4;
  state Lv5
    en:
    VTQD_RegenMode_enum = ENUM_REGENLEVEL_LV5;
    VTQD_SaveRegenMode_enum = ENUM_REGENLEVEL_LV5;
  state One_Pedal_Drive_Mode
    en:
    VTQD_RegenMode_enum = ENUM_REGENLEVEL_OPD;
    VTQD_SaveRegenMode_enum = ENUM_REGENLEVEL_OPD;
  (default) -> OFF : {
      | VTQD_SaveRegenMode_enum = VTQD_ReadRegenMode_enum;
      | }
  Lv1 -> (junction 102) [order 3] : [(VTQD_RegenSWSta_enum == ...
      | ENUM_REGENSWSTA_LONGPRESSUP || ...
      | VINP_SmartEcoModeSW_flg) && ...
      | !VINP_IVISnowModeCmd_flg]
  (junction 102) -> (junction 85)
  (junction 59) -> Lv1 : [VTQD_SaveRegenMode_enum == ENUM_REGENLEVEL_LV1]
  Lv1 -> UserSetting [order 2] : [VTQD_BCMRgnUserEn_flg]
  (junction 56) -> (junction 59) [order 2]
  UserSetting -> Lv1 [order 6] : [VTQD_ActRgnUserSet_enum == ENUM_RGNMODEUSERSET_LV1]
  Lv1 -> OFF [order 1] : [ VPMM_PowerSta_enum != ENUM_POWERSTA_ON && ...
      |  VPMM_PowerSta_enum != ENUM_POWERSTA_READY ]
  Lv1 -> Lv2 [order 4] : [VTQD_RegenSWSta_enum == ...
      | ENUM_REGENSWSTA_SHORTPRESSUP ]
  Lv2 -> Lv1 [order 3] : [VTQD_RegenSWSta_enum == ...
      | ENUM_REGENSWSTA_SHORTPRESSDOWN]
  (junction 56) -> Lv2 [order 1] : [VTQD_SaveRegenMode_enum == ENUM_REGENLEVEL_LV2]
  Lv2 -> (junction 85) [order 4] : [(VTQD_RegenSWSta_enum == ...
      | ENUM_REGENSWSTA_LONGPRESSUP || ...
      | VINP_SmartEcoModeSW_flg) &&...
      | !VINP_IVISnowModeCmd_flg]
  (junction 53) -> (junction 56) [order 2]
  (junction 85) -> (junction 90)
  Lv2 -> UserSetting [order 2] : [VTQD_BCMRgnUserEn_flg]
  Lv2 -> OFF [order 1] : [ VPMM_PowerSta_enum != ENUM_POWERSTA_ON && ...
      |  VPMM_PowerSta_enum != ENUM_POWERSTA_READY ]
  UserSetting -> Lv2 [order 5] : [VTQD_ActRgnUserSet_enum == ENUM_RGNMODEUSERSET_LV2]
  Lv2 -> Lv3 [order 5] : [VTQD_RegenSWSta_enum == ...
      | ENUM_REGENSWSTA_SHORTPRESSUP && ...
      | !VINP_IVISnowModeCmd_flg]
  Lv3 -> Lv2 [order 3] : [VTQD_RegenSWSta_enum == ...
      | ENUM_REGENSWSTA_SHORTPRESSDOWN || ...
      | VINP_IVISnowModeCmd_flg]
  (junction 53) -> Lv3 [order 1] : [VTQD_SaveRegenMode_enum == ENUM_REGENLEVEL_LV3]
  (junction 50) -> (junction 53) [order 2]
  Lv3 -> (junction 90) [order 4] : [(VTQD_RegenSWSta_enum == ...
      | ENUM_REGENSWSTA_LONGPRESSUP || ...
      | VINP_SmartEcoModeSW_flg) && ...
      | !VINP_IVISnowModeCmd_flg]
  (junction 90) -> (junction 95)
  Lv3 -> UserSetting [order 2] : [VTQD_BCMRgnUserEn_flg]
  Lv3 -> OFF [order 1] : [ VPMM_PowerSta_enum != ENUM_POWERSTA_ON && ...
      |  VPMM_PowerSta_enum != ENUM_POWERSTA_READY ]
  UserSetting -> Lv3 [order 4] : [VTQD_ActRgnUserSet_enum == ENUM_RGNMODEUSERSET_LV3]
  Lv3 -> Lv4 [order 5] : [VTQD_RegenSWSta_enum == ...
      | ENUM_REGENSWSTA_SHORTPRESSUP && ...
      | !VINP_IVISnowModeCmd_flg]
  Lv4 -> Lv3 [order 3] : [VTQD_RegenSWSta_enum == ...
      | ENUM_REGENSWSTA_SHORTPRESSDOWN || ...
      | VINP_IVISnowModeCmd_flg]
  (junction 50) -> Lv4 [order 1] : [VTQD_SaveRegenMode_enum == ENUM_REGENLEVEL_LV4]
  Lv4 -> (junction 95) [order 4] : [(VTQD_RegenSWSta_enum == ...
      | ENUM_REGENSWSTA_LONGPRESSUP|| ...
      | VINP_SmartEcoModeSW_flg) && ...
      | !VINP_IVISnowModeCmd_flg ]
  (junction 47) -> (junction 50) [order 2]
  (junction 95) -> (junction 210)
  Lv4 -> UserSetting [order 2] : [VTQD_BCMRgnUserEn_flg]
  UserSetting -> Lv4 [order 3] : [VTQD_ActRgnUserSet_enum == ENUM_RGNMODEUSERSET_LV4]
  Lv4 -> OFF [order 1] : [ VPMM_PowerSta_enum != ENUM_POWERSTA_ON && ...
      |  VPMM_PowerSta_enum != ENUM_POWERSTA_READY ]
  Lv4 -> Lv5 [order 5] : [VTQD_RegenSWSta_enum == ...
      | ENUM_REGENSWSTA_SHORTPRESSUP && ...
      | !VINP_IVISnowModeCmd_flg]
  Lv5 -> Lv4 [order 4] : [VTQD_RegenSWSta_enum == ...
      | ENUM_REGENSWSTA_SHORTPRESSDOWN ||...
      | VINP_IVISnowModeCmd_flg]
  UserSetting -> Lv5 [order 2] : [VTQD_ActRgnUserSet_enum == ENUM_RGNMODEUSERSET_LV5]
  (junction 47) -> Lv5 [order 1] : [VTQD_SaveRegenMode_enum == ENUM_REGENLEVEL_LV5]
  (junction 129) -> (junction 47) [order 2]
  Lv5 -> UserSetting [order 2] : [VTQD_BCMRgnUserEn_flg]
  (junction 210) -> Lv5 [order 1] : [VINP_SmartEcoModeSW_flg && !VINP_IVISnowModeCmd_flg]
  (junction 210) -> (junction 36) [order 2]
  Lv5 -> OFF [order 1] : [ VPMM_PowerSta_enum != ENUM_POWERSTA_ON && ...
      |  VPMM_PowerSta_enum != ENUM_POWERSTA_READY ]
  Lv5 -> (junction 36) [order 3] : [VTQD_RegenSWSta_enum == ...
      | ENUM_REGENSWSTA_LONGPRESSUP && ...
      | !VINP_IVISnowModeCmd_flg && ...
      | !VTQD_TrailerMode_flg && ...
      | !VTQD_OPDModeDis_flg]
      | %add20250215
  (junction 36) -> (junction 39) : [!VTQD_TrailerMode_flg && ...
      |  !VTQD_OPDModeDis_flg]
      | %add20250215
  One_Pedal_Drive_Mode -> Lv5 [order 3] : [VTQD_RegenSWSta_enum == ENUM_REGENSWSTA_SHORTPRESSUP || ...
      |  VTQD_RegenSWSta_enum == ENUM_REGENSWSTA_SHORTPRESSDOWN||...
      |  VINP_IVISnowModeCmd_flg || ...
      |  VTQD_TrailerMode_flg || ...
      |  VTQD_OPDModeDis_flg]
      | %add20250215
  OFF -> (junction 129) [order 2] : [ VPMM_PowerSta_enum == ENUM_POWERSTA_ON || ...
      |  VPMM_PowerSta_enum == ENUM_POWERSTA_READY ]
  (junction 129) -> (junction 205) [order 1]
  OFF -> (junction 220) [order 1] : [VBCM_BCMUserNowSetting_enum != ENUM_BCMUSERNOWSET_INVALID && ...
      |  VBCM_BCMUserNowSetting_enum != ENUM_BCMUSERNOWSET_GUEST && ...
      |  VBCM_BCMUserNowSetting_enum != ENUM_BCMUSERNOWSET_RENT && ...
      |  (VPMM_PowerSta_enum == ENUM_POWERSTA_ON || ...
      |  VPMM_PowerSta_enum == ENUM_POWERSTA_READY)]
      | %add20241217
  (junction 154) -> OFF
  (junction 39) -> One_Pedal_Drive_Mode
  One_Pedal_Drive_Mode -> UserSetting [order 2] : [VTQD_BCMRgnUserEn_flg]
  (junction 205) -> One_Pedal_Drive_Mode : [VTQD_SaveRegenMode_enum == ENUM_REGENLEVEL_OPD]
  One_Pedal_Drive_Mode -> (junction 154) [order 1] : [ VPMM_PowerSta_enum != ENUM_POWERSTA_ON && ...
      |  VPMM_PowerSta_enum != ENUM_POWERSTA_READY ]
  UserSetting -> One_Pedal_Drive_Mode [order 1] : [VTQD_ActRgnUserSet_enum == ENUM_RGNMODEUSERSET_OPD]
  (junction 222) -> UserSetting
  (junction 220) -> (junction 222)
  data: VTQD_RegenMode_enum output uint8 =0; ENUM_REGENLEVEL_LV1 parameter; ENUM_REGENLEVEL_LV2 parameter; ENUM_REGENLEVEL_LV3 parameter; ENUM_REGENLEVEL_LV4 parameter; ENUM_REGENLEVEL_LV5 parameter; ENUM_REGENLEVEL_OPD parameter; VPMM_PowerSta_enum input; ENUM_POWERSTA_ON parameter; ENUM_POWERSTA_READY parameter; VTQD_RegenSWSta_enum input; ENUM_REGENSWSTA_LONGPRESSUP parameter; ENUM_REGENSWSTA_SHORTPRESSDOWN parameter; ENUM_REGENSWSTA_SHORTPRESSUP parameter; ENUM_REGENLEVEL_OFF parameter; VTQD_SaveRegenMode_enum output uint8; VTQD_ReadRegenMode_enum input; VINP_SmartEcoModeSW_flg input; VINP_IVISnowModeCmd_flg input; VTQD_TrailerMode_flg input; VTQD_BCMRgnUserEn_flg input; VTQD_ActRgnUserSet_enum input; VBCM_BCMUserNowSetting_enum input; ENUM_BCMUSERNOWSET_INVALID parameter; ENUM_BCMUSERNOWSET_GUEST parameter; ENUM_BCMUSERNOWSET_RENT parameter; ENUM_RGNMODEUSERSET_LV1 parameter; ENUM_RGNMODEUSERSET_LV2 parameter; ENUM_RGNMODEUSERSET_LV3 parameter; ENUM_RGNMODEUSERSET_LV4 parameter; ENUM_RGNMODEUSERSET_LV5 parameter; ENUM_RGNMODEUSERSET_OPD parameter; VTQD_OPDModeDis_flg input
